simulink model "Translational_system"  (R2023b)
settings: Solver=VariableStepAuto  StartTime=0.0  StopTime=10.0  RelTol=1e-3
undefined symbols (not defined in the file): Cx, Kx, m1, m2
settings Model: Creator=Santhosh  LastModifiedBy=Santhosh

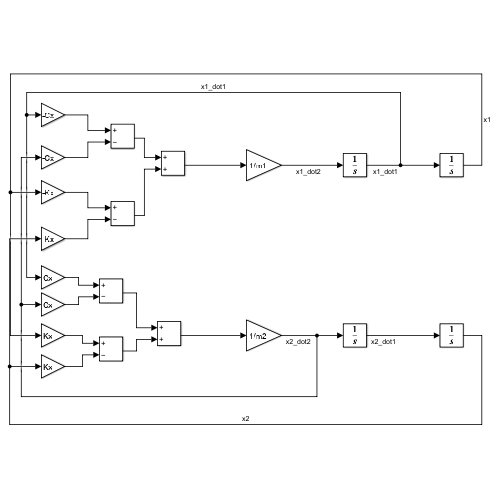
[thumbnail: Simulink's stored preview of the top-level diagram]
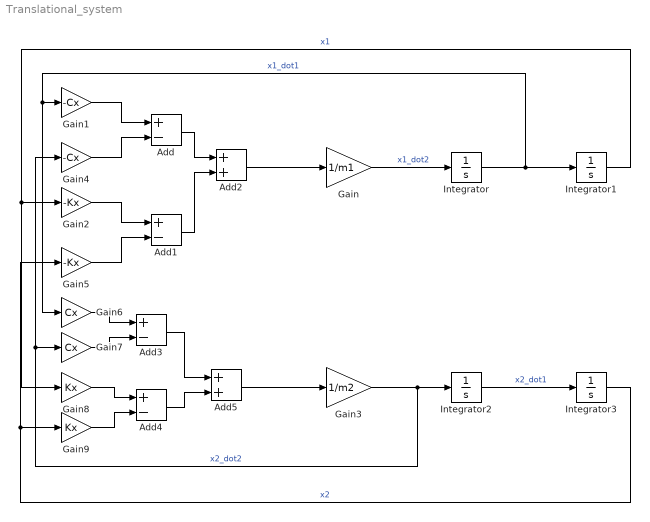
== system Translational_system ==
  Add{,1,3..4} (4 alike) : Sum  Inputs=+-
  Add2 : Sum
  Add5 : Sum
  Gain : Gain  Gain=1/m1
  Gain1 : Gain  Gain=-Cx
  Gain2 : Gain  Gain=-Kx
  Gain3 : Gain  Gain=1/m2
  Gain4 : Gain  Gain=-Cx
  Gain5 : Gain  Gain=-Kx
  Gain6 : Gain  Gain=Cx
  Gain7 : Gain  Gain=Cx
  Gain8 : Gain  Gain=Kx
  Gain9 : Gain  Gain=Kx
  Integrator{,1..3} (4 alike) : Integrator
  wires:
  Gain/1 -> Integrator/1  "x1_dot2"
  Integrator/1 -> Gain6/1, Gain1/1, Integrator1/1  "x1_dot1"
  Gain3/1 -> Gain7/1, Gain4/1, Integrator2/1  "x2_dot2"
  Integrator2/1 -> Integrator3/1  "x2_dot1"
  Integrator1/1 -> Gain2/1, Gain8/1  "x1"
  Gain1/1 -> Add/1
  Gain4/1 -> Add/2
  Gain2/1 -> Add1/1
  Gain5/1 -> Add1/2
  Add/1 -> Add2/1
  Add1/1 -> Add2/2
  Add2/1 -> Gain/1
  Integrator3/1 -> Gain9/1, Gain5/1  "x2"
  Gain6/1 -> Add3/1
  Gain7/1 -> Add3/2
  Gain8/1 -> Add4/1
  Gain9/1 -> Add4/2
  Add3/1 -> Add5/1
  Add4/1 -> Add5/2
  Add5/1 -> Gain3/1
